simulink model "ex8_planar_robot_ct_disturbance_esti_simulation"  (R2016b)
settings: Solver=FixedStepAuto  StartTime=0.0  StopTime=10  FixedStep=0.001  RelTol=1e-3  EnableMultiTasking=on
values from neighbouring files (symbols this model uses):
  a1 = u_gen(15)    [classical_joint_planar_robot_simulink.m]    (also in ct_gravit_planar_robot_simulink.m = u_gen(13); ct_pid_planar_robot_simulink.m; ct_planar_robot_simulink.m = u_gen(13); ex_planar_robot_2dof.m = 1)
  a2 = u_gen(16)    [classical_joint_planar_robot_simulink.m]    (also in ct_gravit_planar_robot_simulink.m = u_gen(14); ct_pid_planar_robot_simulink.m; ct_planar_robot_simulink.m = u_gen(14); ex_planar_robot_2dof.m = 1)
  g = u_gen(17)    [classical_joint_planar_robot_simulink.m]    (also in ct_gravit_planar_robot_simulink.m; ct_pid_planar_robot_simulink.m; ct_planar_robot_simulink.m = u_gen(15); ex_planar_robot_2dof.m = 9.81)
  kp1 = wn1^2    [ex_planar_robot_2dof.m]
  kp2 = wn2^2    [ex_planar_robot_2dof.m]
  kv1 = 100    [ex_planar_robot_2dof.m]
  kv2 = 100    [ex_planar_robot_2dof.m]
  l1 = 100    [ex_planar_robot_2dof.m]
  l2 = 100    [ex_planar_robot_2dof.m]
  m1 = u_gen(11)    [ac_controller_simulink.m]    (also in classical_joint_planar_robot_simulink.m = u_gen(13); ct_gravit_planar_robot_simulink.m; ct_pid_planar_robot_simulink.m = u_gen(13); ct_planar_robot_simulink.m)
  M11 = eval((subs(M(1,1), q2, 0) + subs(M(1,1), q2, pi)))/2    [ex_planar_robot_2dof.m]
  m2 = u_gen(12)    [ac_controller_simulink.m]    (also in classical_joint_planar_robot_simulink.m = u_gen(14); ct_gravit_planar_robot_simulink.m; ct_pid_planar_robot_simulink.m = u_gen(14); ct_planar_robot_simulink.m)
  M22 = eval(M(2,2))    [ex_planar_robot_2dof.m]
settings Model: Creator=sevimeda  LastModifiedBy=kargto
settings OptimizationCC: LifeSpan=inf
settings DebuggingCC: SFUnexpectedBacktrackingDiag=warning  SFNoUnconditionalDefaultTransitionDiag=warning  SFExecutionAtInitializationDiag=none
settings GRTTargetCC: TargetLangStandard=C89/C90 (ANSI)  GeneratePreprocessorConditionals=Disable all
settings ConfigComp: CovMetricSettings=dw  CovHtmlReporting=on  CovSaveCumulativeToWorkspaceVar=on  CovSaveSingleToWorkspaceVar=on  CovExternalEMLEnable=off

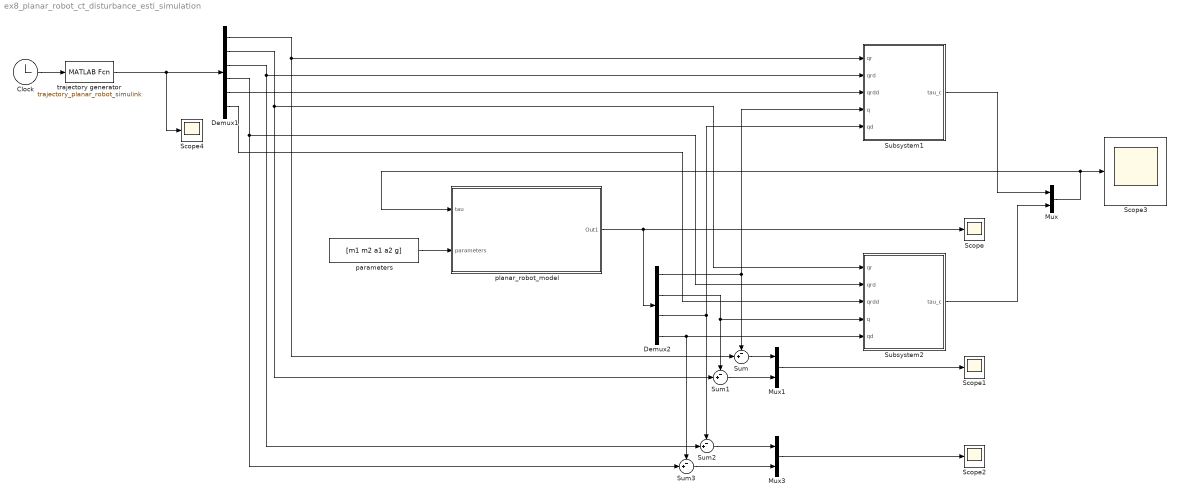
== system ex8_planar_robot_ct_disturbance_esti_simulation ==
  Clock : Clock
  Demux1 : Demux  Outputs=6
  Demux2 : Demux
  Mux : Mux  Inputs=2
  Mux1 : Mux  Inputs=2
  Mux3 : Mux  Inputs=2
  Scope{,1..4} (5 alike) : Scope
  Subsystem1 : Subsystem
  Subsystem2 : Subsystem
  Sum{,1..3} (4 alike) : Sum  Inputs=-+|
  parameters : Constant  Value=[m1 m2 a1 a2 g]
  planar_robot_model : Subsystem
  trajectory generator : MATLABFcn  MATLABFcn=trajectory_planar_robot_simulink
  wires:
  Clock/1 -> trajectory generator/1
  trajectory generator/1 -> Scope4/1, Demux1/1
  parameters/1 -> planar_robot_model/2(parameters)
  planar_robot_model/1(Out1) -> Scope/1, Demux2/1
  Demux1/1 -> Sum/2, Subsystem1/1(qr)
  Demux2/1 -> Subsystem1/4(q), Sum/1
  Sum/1 -> Mux1/1
  Demux2/2 -> Sum1/1, Subsystem2/4(q)
  Sum1/1 -> Mux1/2
  Demux1/2 -> Subsystem2/1(qr), Sum1/2
  Sum2/1 -> Mux3/1
  Sum3/1 -> Mux3/2
  Demux2/3 -> Subsystem1/5(qd), Sum2/1
  Demux2/4 -> Sum3/1, Subsystem2/5(qd)
  Demux1/3 -> Sum2/2, Subsystem1/2(qrd)
  Demux1/4 -> Subsystem2/2(qrd), Sum3/2
  Mux1/1 -> Scope1/1
  Mux3/1 -> Scope2/1
  Demux1/5 -> Subsystem1/3(qrdd)
  Demux1/6 -> Subsystem2/3(qrdd)
  Subsystem1/1(tau_c) -> Mux/1
  Subsystem2/1(tau_c) -> Mux/2
  Mux/1 -> planar_robot_model/1(tau), Scope3/1

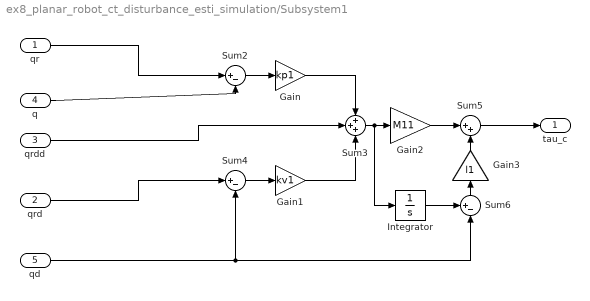
== system ex8_planar_robot_ct_disturbance_esti_simulation/Subsystem1 ==
  qr : Inport
  qrd : Inport  Port=2
  qrdd : Inport  Port=3
  q : Inport  Port=4
  qd : Inport  Port=5
  Gain : Gain  Gain=kp1
  Gain1 : Gain  Gain=kv1
  Gain2 : Gain  Gain=M11
  Gain3 : Gain  Gain=l1
  Integrator : Integrator
  Sum2 : Sum  Inputs=|+-
  Sum3 : Sum  Inputs=+++
  Sum4 : Sum  Inputs=|+-
  Sum5 : Sum  Inputs=|++
  Sum6 : Sum  Inputs=+-|
  tau_c : Outport
  wires:
  qd/1 -> Sum6/2, Sum4/2
  qrd/1 -> Sum4/1
  qr/1 -> Sum2/1
  Sum6/1 -> Gain3/1
  qrdd/1 -> Sum3/2
  Integrator/1 -> Sum6/1
  Gain1/1 -> Sum3/3
  q/1 -> Sum2/2
  Gain3/1 -> Sum5/2
  Sum2/1 -> Gain/1
  Gain/1 -> Sum3/1
  Sum5/1 -> tau_c/1
  Gain2/1 -> Sum5/1
  Sum3/1 -> Gain2/1, Integrator/1
  Sum4/1 -> Gain1/1

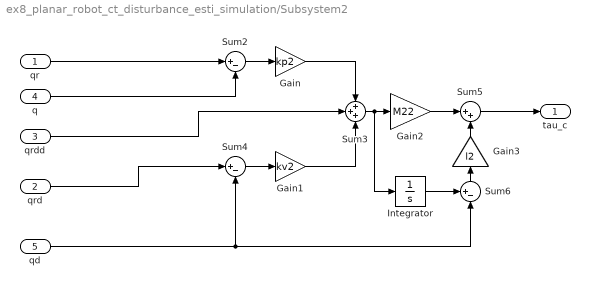
== system ex8_planar_robot_ct_disturbance_esti_simulation/Subsystem2 ==
  qr : Inport
  qrd : Inport  Port=2
  qrdd : Inport  Port=3
  q : Inport  Port=4
  qd : Inport  Port=5
  Gain : Gain  Gain=kp2
  Gain1 : Gain  Gain=kv2
  Gain2 : Gain  Gain=M22
  Gain3 : Gain  Gain=l2
  Integrator : Integrator
  Sum2 : Sum  Inputs=|+-
  Sum3 : Sum  Inputs=+++
  Sum4 : Sum  Inputs=|+-
  Sum5 : Sum  Inputs=|++
  Sum6 : Sum  Inputs=+-|
  tau_c : Outport
  wires:
  qd/1 -> Sum6/2, Sum4/2
  qrd/1 -> Sum4/1
  qr/1 -> Sum2/1
  Sum6/1 -> Gain3/1
  qrdd/1 -> Sum3/2
  Integrator/1 -> Sum6/1
  Gain1/1 -> Sum3/3
  q/1 -> Sum2/2
  Gain3/1 -> Sum5/2
  Sum2/1 -> Gain/1
  Gain/1 -> Sum3/1
  Sum5/1 -> tau_c/1
  Gain2/1 -> Sum5/1
  Sum3/1 -> Gain2/1, Integrator/1
  Sum4/1 -> Gain1/1

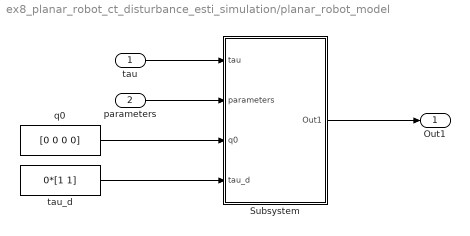
== system ex8_planar_robot_ct_disturbance_esti_simulation/planar_robot_model ==
  tau : Inport
  parameters : Inport  Port=2
  Subsystem : Subsystem
  q0 : Constant  Value=[0 0 0 0]
  tau_d : Constant  Value=0*[1 1]
  Out1 : Outport
  wires:
  Subsystem/1(Out1) -> Out1/1
  q0/1 -> Subsystem/3(q0)
  tau_d/1 -> Subsystem/4(tau_d)
  tau/1 -> Subsystem/1(tau)
  parameters/1 -> Subsystem/2(parameters)

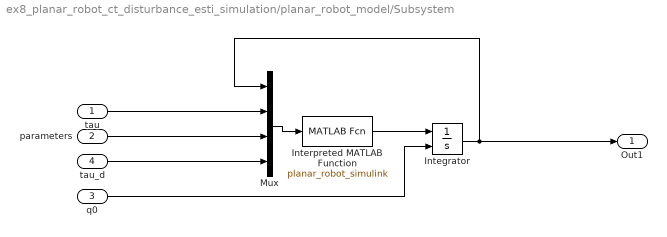
== system ex8_planar_robot_ct_disturbance_esti_simulation/planar_robot_model/Subsystem ==
  tau : Inport
  parameters : Inport  Port=2
  q0 : Inport  Port=3
  tau_d : Inport  Port=4
  Integrator : Integrator  InitialConditionSource=external
  Interpreted MATLAB Function : MATLABFcn  MATLABFcn=planar_robot_simulink  OutputDimensions=4
  Mux : Mux
  Out1 : Outport
  wires:
  Interpreted MATLAB Function/1 -> Integrator/1
  q0/1 -> Integrator/2
  Mux/1 -> Interpreted MATLAB Function/1
  Integrator/1 -> Out1/1, Mux/1
  tau/1 -> Mux/2
  parameters/1 -> Mux/3
  tau_d/1 -> Mux/4
